simulink library "sudoku_lib"  (R2018b)
settings: Solver=VariableStepAuto  StartTime=0.0  StopTime=10.0  RelTol=1e-3
libraries: $bdroot x28
settings Model: Creator=F074018  LastModifiedBy=F074018

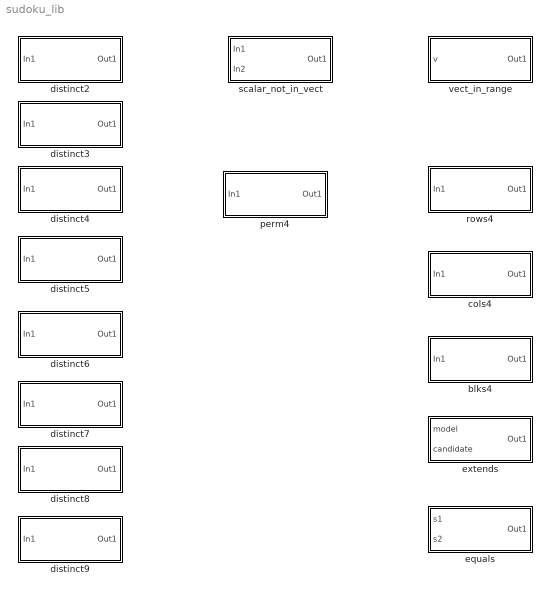
== system sudoku_lib ==
  blks4 : Subsystem
  cols4 : Subsystem
  distinct2 : Subsystem
  distinct3 : Subsystem
  distinct4 : Subsystem
  distinct5 : Subsystem
  distinct6 : Subsystem
  distinct7 : Subsystem
  distinct8 : Subsystem
  distinct9 : Subsystem
  equals : Subsystem
  extends : Subsystem
  perm4 : Subsystem
  rows4 : Subsystem
  scalar_not_in_vect : Subsystem
  vect_in_range : Subsystem

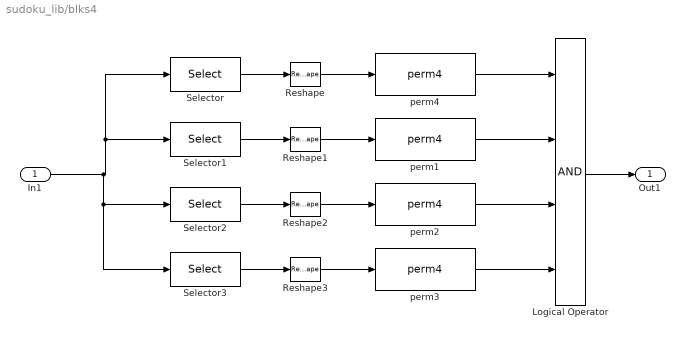
== system sudoku_lib/blks4 ==
  In1 : Inport  PortDimensions=[4 4]
      settings: AttributesFormatString=%<PortDimensions>
  Logical Operator : Logic  Inputs=4  AllPortsSameDT=off  OutDataTypeStr=boolean
  Reshape{,1..3} (4 alike) : Reshape
  Selector : Selector  NumberOfDimensions=2  InputPortWidth=3  IndexOptions=Index vector (dialog),Index vector (dialog)  Indices=1:2,1:2  OutputSizes=1,1
      settings: AttributesFormatString=|
      | %<IndexOptions>
      | %<Indices>
  Selector1 : Selector  NumberOfDimensions=2  InputPortWidth=3  IndexOptions=Index vector (dialog),Index vector (dialog)  Indices=1:2,3:4  OutputSizes=1,1
      settings: AttributesFormatString=|
      | %<IndexOptions>
      | %<Indices>
  Selector2 : Selector  NumberOfDimensions=2  InputPortWidth=3  IndexOptions=Index vector (dialog),Index vector (dialog)  Indices=3:4,1:2  OutputSizes=1,1
      settings: AttributesFormatString=|
      | %<IndexOptions>
      | %<Indices>
  Selector3 : Selector  NumberOfDimensions=2  InputPortWidth=3  IndexOptions=Index vector (dialog),Index vector (dialog)  Indices=3:4,3:4  OutputSizes=1,1
      settings: AttributesFormatString=|
      | %<IndexOptions>
      | %<Indices>
  perm{1..4} (4 alike) : $bdroot/perm4  SystemSampleTime=-1
  Out1 : Outport
  wires:
  Logical Operator/1 -> Out1/1
  perm4/1 -> Logical Operator/1
  perm1/1 -> Logical Operator/2
  perm2/1 -> Logical Operator/3
  perm3/1 -> Logical Operator/4
  In1/1 -> Selector2/1, Selector3/1, Selector/1, Selector1/1
  Selector/1 -> Reshape/1
  Selector1/1 -> Reshape1/1
  Selector2/1 -> Reshape2/1
  Selector3/1 -> Reshape3/1
  Reshape/1 -> perm4/1
  Reshape1/1 -> perm1/1
  Reshape2/1 -> perm2/1
  Reshape3/1 -> perm3/1

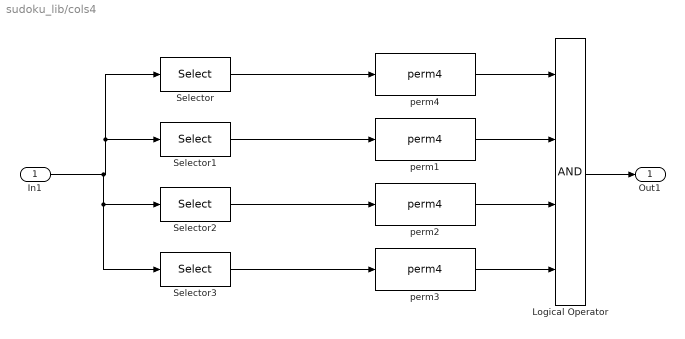
== system sudoku_lib/cols4 ==
  In1 : Inport  PortDimensions=[4 4]
      settings: AttributesFormatString=%<PortDimensions>
  Logical Operator : Logic  Inputs=4  AllPortsSameDT=off  OutDataTypeStr=boolean
  Selector : Selector  NumberOfDimensions=2  InputPortWidth=3  IndexOptions=Select all,Index vector (dialog)  Indices=1,1  OutputSizes=1,1
      settings: AttributesFormatString=|
      | %<IndexOptions>
      | %<Indices>
  Selector1 : Selector  NumberOfDimensions=2  InputPortWidth=3  IndexOptions=Select all,Index vector (dialog)  Indices=1,2  OutputSizes=1,1
      settings: AttributesFormatString=|
      | %<IndexOptions>
      | %<Indices>
  Selector2 : Selector  NumberOfDimensions=2  InputPortWidth=3  IndexOptions=Select all,Index vector (dialog)  Indices=1,3  OutputSizes=1,1
      settings: AttributesFormatString=|
      | %<IndexOptions>
      | %<Indices>
  Selector3 : Selector  NumberOfDimensions=2  InputPortWidth=3  IndexOptions=Select all,Index vector (dialog)  Indices=1,4  OutputSizes=1,1
      settings: AttributesFormatString=|
      | %<IndexOptions>
      | %<Indices>
  perm{1..4} (4 alike) : $bdroot/perm4  SystemSampleTime=-1
  Out1 : Outport
  wires:
  Logical Operator/1 -> Out1/1
  perm4/1 -> Logical Operator/1
  perm1/1 -> Logical Operator/2
  perm2/1 -> Logical Operator/3
  perm3/1 -> Logical Operator/4
  In1/1 -> Selector2/1, Selector3/1, Selector/1, Selector1/1
  Selector/1 -> perm4/1
  Selector1/1 -> perm1/1
  Selector2/1 -> perm2/1
  Selector3/1 -> perm3/1

== system sudoku_lib/distinct2 ==
  In1 : Inport
  Demux : Demux  Outputs=[1 1]
      settings: AttributesFormatString=%<Outputs>
  Relational Operator : RelationalOperator  Operator=~=  OutDataTypeStr=boolean  RndMeth=Simplest  InputSameDT=on
  Out1 : Outport
  wires:
  In1/1 -> Demux/1
  Relational Operator/1 -> Out1/1
  Demux/1 -> Relational Operator/1
  Demux/2 -> Relational Operator/2

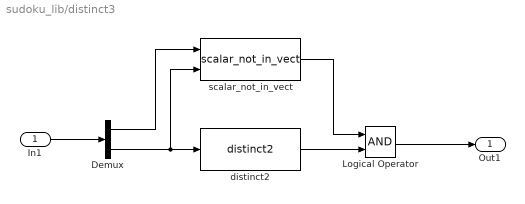
== system sudoku_lib/distinct3 ==
  In1 : Inport
  Demux : Demux  Outputs=[1 2]
      settings: AttributesFormatString=%<Outputs>
  Logical Operator : Logic  OutDataTypeStr=boolean
  distinct2 : $bdroot/distinct2  SystemSampleTime=-1
  scalar_not_in_vect : $bdroot/scalar_not_in_vect  SystemSampleTime=-1
  Out1 : Outport
  wires:
  In1/1 -> Demux/1
  Demux/2 -> scalar_not_in_vect/2, distinct2/1
  distinct2/1 -> Logical Operator/2
  Logical Operator/1 -> Out1/1
  Demux/1 -> scalar_not_in_vect/1
  scalar_not_in_vect/1 -> Logical Operator/1

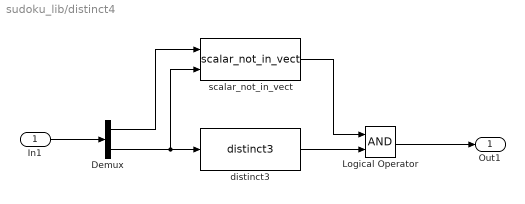
== system sudoku_lib/distinct4 ==
  In1 : Inport
  Demux : Demux  Outputs=[1 3]
      settings: AttributesFormatString=%<Outputs>
  Logical Operator : Logic  OutDataTypeStr=boolean
  distinct3 : $bdroot/distinct3  SystemSampleTime=-1
  scalar_not_in_vect : $bdroot/scalar_not_in_vect  SystemSampleTime=-1
  Out1 : Outport
  wires:
  In1/1 -> Demux/1
  Demux/2 -> distinct3/1, scalar_not_in_vect/2
  distinct3/1 -> Logical Operator/2
  Logical Operator/1 -> Out1/1
  Demux/1 -> scalar_not_in_vect/1
  scalar_not_in_vect/1 -> Logical Operator/1

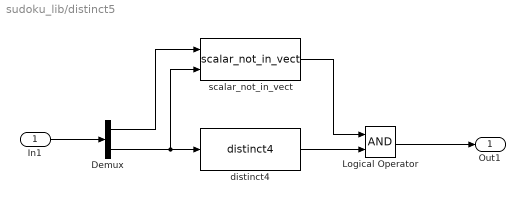
== system sudoku_lib/distinct5 ==
  In1 : Inport
  Demux : Demux  Outputs=[1 4]
      settings: AttributesFormatString=%<Outputs>
  Logical Operator : Logic  OutDataTypeStr=boolean
  distinct4 : $bdroot/distinct4  SystemSampleTime=-1
  scalar_not_in_vect : $bdroot/scalar_not_in_vect  SystemSampleTime=-1
  Out1 : Outport
  wires:
  In1/1 -> Demux/1
  Demux/2 -> distinct4/1, scalar_not_in_vect/2
  distinct4/1 -> Logical Operator/2
  Logical Operator/1 -> Out1/1
  Demux/1 -> scalar_not_in_vect/1
  scalar_not_in_vect/1 -> Logical Operator/1

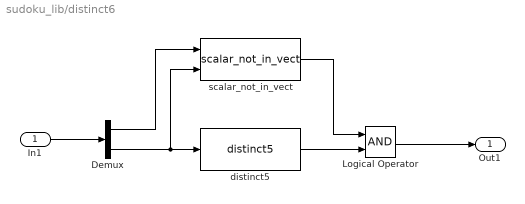
== system sudoku_lib/distinct6 ==
  In1 : Inport
  Demux : Demux  Outputs=[1 5]
      settings: AttributesFormatString=%<Outputs>
  Logical Operator : Logic  OutDataTypeStr=boolean
  distinct5 : $bdroot/distinct5  SystemSampleTime=-1
  scalar_not_in_vect : $bdroot/scalar_not_in_vect  SystemSampleTime=-1
  Out1 : Outport
  wires:
  In1/1 -> Demux/1
  Demux/2 -> distinct5/1, scalar_not_in_vect/2
  distinct5/1 -> Logical Operator/2
  Logical Operator/1 -> Out1/1
  Demux/1 -> scalar_not_in_vect/1
  scalar_not_in_vect/1 -> Logical Operator/1

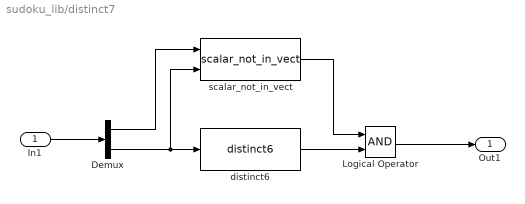
== system sudoku_lib/distinct7 ==
  In1 : Inport
  Demux : Demux  Outputs=[1 6]
      settings: AttributesFormatString=%<Outputs>
  Logical Operator : Logic  OutDataTypeStr=boolean
  distinct6 : $bdroot/distinct6  SystemSampleTime=-1
  scalar_not_in_vect : $bdroot/scalar_not_in_vect  SystemSampleTime=-1
  Out1 : Outport
  wires:
  In1/1 -> Demux/1
  Demux/2 -> distinct6/1, scalar_not_in_vect/2
  distinct6/1 -> Logical Operator/2
  Logical Operator/1 -> Out1/1
  Demux/1 -> scalar_not_in_vect/1
  scalar_not_in_vect/1 -> Logical Operator/1

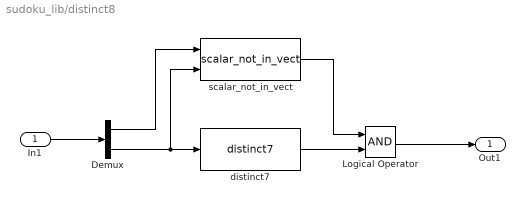
== system sudoku_lib/distinct8 ==
  In1 : Inport
  Demux : Demux  Outputs=[1 7]
      settings: AttributesFormatString=%<Outputs>
  Logical Operator : Logic  OutDataTypeStr=boolean
  distinct7 : $bdroot/distinct7  SystemSampleTime=-1
  scalar_not_in_vect : $bdroot/scalar_not_in_vect  SystemSampleTime=-1
  Out1 : Outport
  wires:
  In1/1 -> Demux/1
  Demux/2 -> distinct7/1, scalar_not_in_vect/2
  distinct7/1 -> Logical Operator/2
  Logical Operator/1 -> Out1/1
  Demux/1 -> scalar_not_in_vect/1
  scalar_not_in_vect/1 -> Logical Operator/1

== system sudoku_lib/distinct9 ==
  In1 : Inport
  Demux : Demux  Outputs=[1 8]
      settings: AttributesFormatString=%<Outputs>
  Logical Operator : Logic  OutDataTypeStr=boolean
  distinct8 : $bdroot/distinct8  SystemSampleTime=-1
  scalar_not_in_vect : $bdroot/scalar_not_in_vect  SystemSampleTime=-1
  Out1 : Outport
  wires:
  In1/1 -> Demux/1
  Demux/2 -> distinct8/1, scalar_not_in_vect/2
  distinct8/1 -> Logical Operator/2
  Logical Operator/1 -> Out1/1
  Demux/1 -> scalar_not_in_vect/1
  scalar_not_in_vect/1 -> Logical Operator/1

== system sudoku_lib/equals ==
  s1 : Inport
  s2 : Inport  Port=2
  Logical Operator2 : Logic  Inputs=1  OutDataTypeStr=boolean
  Relational Operator1 : RelationalOperator  Operator===  OutDataTypeStr=boolean  RndMeth=Simplest  InputSameDT=on
  Reshape : Reshape
  Out1 : Outport  PortDimensions=1
  wires:
  s1/1 -> Relational Operator1/1
  s2/1 -> Relational Operator1/2
  Relational Operator1/1 -> Reshape/1
  Reshape/1 -> Logical Operator2/1
  Logical Operator2/1 -> Out1/1

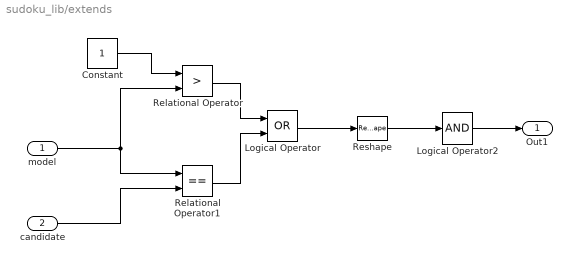
== system sudoku_lib/extends ==
  model : Inport
  candidate : Inport  Port=2
  Constant : Constant
  Logical Operator : Logic  Operator=OR  OutDataTypeStr=boolean
  Logical Operator2 : Logic  Inputs=1  OutDataTypeStr=boolean
  Relational Operator : RelationalOperator  Operator=>  OutDataTypeStr=boolean  RndMeth=Simplest
  Relational Operator1 : RelationalOperator  Operator===  OutDataTypeStr=boolean  RndMeth=Simplest
  Reshape : Reshape
  Out1 : Outport  PortDimensions=1
  wires:
  model/1 -> Relational Operator/2, Relational Operator1/1
  Constant/1 -> Relational Operator/1
  candidate/1 -> Relational Operator1/2
  Relational Operator/1 -> Logical Operator/1
  Relational Operator1/1 -> Logical Operator/2
  Logical Operator/1 -> Reshape/1
  Reshape/1 -> Logical Operator2/1
  Logical Operator2/1 -> Out1/1

== system sudoku_lib/perm4 ==
  In1 : Inport
  Logical Operator : Logic  AllPortsSameDT=off  OutDataTypeStr=boolean
  distinct4 : $bdroot/distinct4  SystemSampleTime=-1
  vect_in_range : $bdroot/vect_in_range  SystemSampleTime=-1
  Out1 : Outport
  wires:
  In1/1 -> distinct4/1, vect_in_range/1
  vect_in_range/1 -> Logical Operator/1
  distinct4/1 -> Logical Operator/2
  Logical Operator/1 -> Out1/1

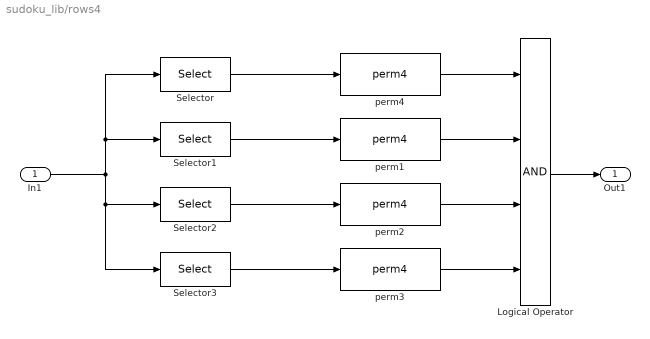
== system sudoku_lib/rows4 ==
  In1 : Inport  PortDimensions=[4 4]
      settings: AttributesFormatString=%<PortDimensions>
  Logical Operator : Logic  Inputs=4  AllPortsSameDT=off  OutDataTypeStr=boolean
  Selector : Selector  NumberOfDimensions=2  InputPortWidth=3  IndexOptions=Index vector (dialog),Select all  Indices=1,1  OutputSizes=1,1
      settings: AttributesFormatString=|
      | %<IndexOptions>
      | %<Indices>
  Selector1 : Selector  NumberOfDimensions=2  InputPortWidth=3  IndexOptions=Index vector (dialog),Select all  Indices=2,1  OutputSizes=1,1
      settings: AttributesFormatString=|
      | %<IndexOptions>
      | %<Indices>
  Selector2 : Selector  NumberOfDimensions=2  InputPortWidth=3  IndexOptions=Index vector (dialog),Select all  Indices=3,1  OutputSizes=1,1
      settings: AttributesFormatString=|
      | %<IndexOptions>
      | %<Indices>
  Selector3 : Selector  NumberOfDimensions=2  InputPortWidth=3  IndexOptions=Index vector (dialog),Select all  Indices=4,1  OutputSizes=1,1
      settings: AttributesFormatString=|
      | %<IndexOptions>
      | %<Indices>
  perm{1..4} (4 alike) : $bdroot/perm4  SystemSampleTime=-1
  Out1 : Outport
  wires:
  Logical Operator/1 -> Out1/1
  perm4/1 -> Logical Operator/1
  perm1/1 -> Logical Operator/2
  perm2/1 -> Logical Operator/3
  perm3/1 -> Logical Operator/4
  In1/1 -> Selector2/1, Selector3/1, Selector1/1, Selector/1
  Selector/1 -> perm4/1
  Selector1/1 -> perm1/1
  Selector2/1 -> perm2/1
  Selector3/1 -> perm3/1

== system sudoku_lib/scalar_not_in_vect ==
  In1 : Inport  PortDimensions=1
  In2 : Inport  Port=2
  Logical Operator : Logic  Inputs=1  OutDataTypeStr=boolean
  Relational Operator : RelationalOperator  Operator=~=  OutDataTypeStr=boolean  RndMeth=Simplest  InputSameDT=on
  Out1 : Outport
  wires:
  In2/1 -> Relational Operator/2
  In1/1 -> Relational Operator/1
  Relational Operator/1 -> Logical Operator/1
  Logical Operator/1 -> Out1/1

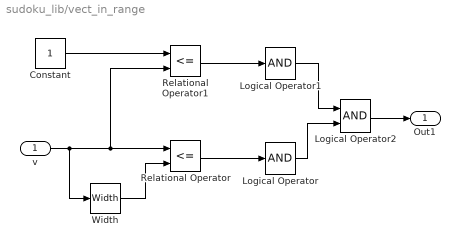
== system sudoku_lib/vect_in_range ==
  v : Inport
  Constant : Constant
  Logical Operator : Logic  Inputs=1  OutDataTypeStr=boolean
  Logical Operator1 : Logic  Inputs=1  OutDataTypeStr=boolean
  Logical Operator2 : Logic  OutDataTypeStr=boolean
  Relational Operator : RelationalOperator  Operator=<=  OutDataTypeStr=boolean  RndMeth=Simplest
  Relational Operator1 : RelationalOperator  Operator=<=  OutDataTypeStr=boolean  RndMeth=Simplest
  Width : Width
  Out1 : Outport
  wires:
  v/1 -> Width/1, Relational Operator1/2, Relational Operator/1
  Relational Operator/1 -> Logical Operator/1
  Constant/1 -> Relational Operator1/1
  Relational Operator1/1 -> Logical Operator1/1
  Logical Operator1/1 -> Logical Operator2/1
  Logical Operator/1 -> Logical Operator2/2
  Logical Operator2/1 -> Out1/1
  Width/1 -> Relational Operator/2
